simulink model "firstmodel"  (R2025a)
settings: Solver=FixedStepAuto  StartTime=0.0  StopTime=1  FixedStep=0.001  RelTol=1e-3
undefined symbols (not defined in the file): DiscIntNeverNeededParam
settings Model: Creator=DELL  LastModifiedBy=DELL

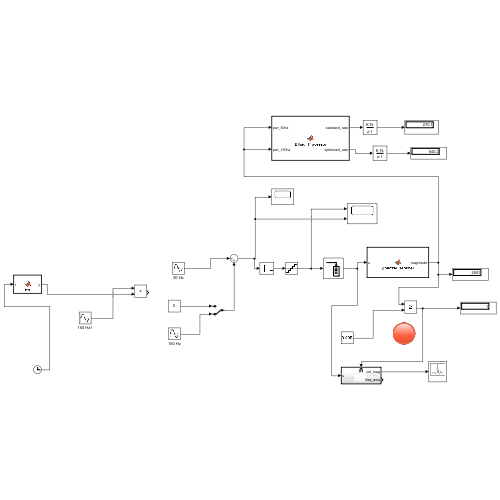
[thumbnail: Simulink's stored preview of the top-level diagram]
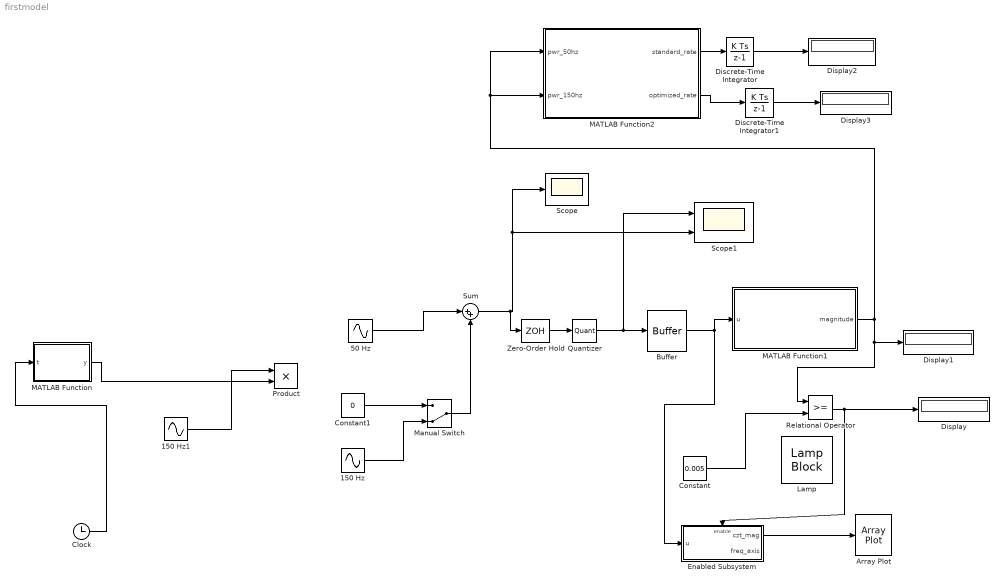
== system firstmodel ==
  150 Hz : Sin  Frequency=300*pi  SampleTime=0
  150 Hz1 : Sin  Frequency=300*pi  SampleTime=0
  50 Hz : Sin  Frequency=100*pi  SampleTime=0
  Array Plot : ArrayPlot  WindowPosition=[134.000000,171.000000,800.000000,500.000000,]  ScopeFrameLocation=window  SampleIncrement=0.02  XOffset=140  YLimits=[3.4950518655331093 6.194518570220462]
      settings: OpenAtSimulationStart=off
  Buffer : Buffer  N=100  OutputFrames=off
  Clock : Clock
  Constant : Constant  Value=0.005
  Constant1 : Constant  Value=0
  Discrete-Time Integrator : DiscreteIntegrator  SampleTime=-1  ICPrevOutput=DiscIntNeverNeededParam  ICPrevScaledInput=DiscIntNeverNeededParam
  Discrete-Time Integrator1 : DiscreteIntegrator  SampleTime=-1  ICPrevOutput=DiscIntNeverNeededParam  ICPrevScaledInput=DiscIntNeverNeededParam
  Display{,1..3} (4 alike) : Display
  Enabled Subsystem : Subsystem  TreatAsAtomicUnit=on
  Lamp : LampBlock  LabelPosition=Hide  DefaultColor=[192.0, 192.0, 192.0]
  MATLAB Function : MATLAB Function  TreatAsAtomicUnit=on
  MATLAB Function1 : MATLAB Function  TreatAsAtomicUnit=on
  MATLAB Function2 : MATLAB Function  TreatAsAtomicUnit=on
  Manual Switch : ManualSwitch  CurrentSetting=0
  Product : Product
  Quantizer : Quantizer  QuantizationInterval=2/4096
  Relational Operator : RelationalOperator  OutDataTypeStr=boolean  RndMeth=Simplest  InputSameDT=off
  Scope : Scope
      settings: ActiveDisplayYMinimum=-1.6931778606615959  ActiveDisplayYMaximum=1.933966715724176
  Scope1 : Scope  NumInputPorts=2
      settings: ActiveDisplayYMinimum=-1.923828125  ActiveDisplayYMaximum=1.923828125
  Sum : Sum  Inputs=|++
  Zero-Order Hold : ZeroOrderHold  SampleTime=1/1000
  wires:
  50 Hz/1 -> Sum/1
  Sum/1 -> Scope/1, Scope1/2, Zero-Order Hold/1
  Clock/1 -> MATLAB Function/1(t)
  MATLAB Function/1(y) -> Product/2
  Zero-Order Hold/1 -> Quantizer/1
  Quantizer/1 -> Buffer/1, Scope1/1
  Buffer/1 -> Enabled Subsystem/1(u), MATLAB Function1/1(u)
  MATLAB Function1/1(magnitude) -> MATLAB Function2/2(pwr_150hz), MATLAB Function2/1(pwr_50hz), Display1/1, Relational Operator/1
  Constant/1 -> Relational Operator/2
  Relational Operator/1 -> Display/1, Enabled Subsystem/Enable
  Constant1/1 -> Manual Switch/1
  150 Hz/1 -> Manual Switch/2
  Enabled Subsystem/1(czt_mag) -> Array Plot/1
  150 Hz1/1 -> Product/1
  MATLAB Function2/1(standard_rate) -> Discrete-Time Integrator/1
  Manual Switch/1 -> Sum/2
  MATLAB Function2/2(optimized_rate) -> Discrete-Time Integrator1/1
  Discrete-Time Integrator/1 -> Display2/1
  Discrete-Time Integrator1/1 -> Display3/1

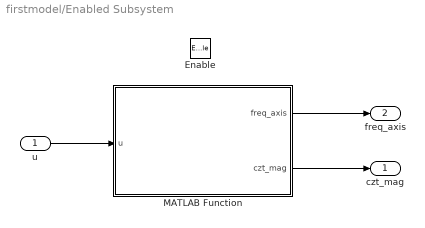
== system firstmodel/Enabled Subsystem ==
  u : Inport
  Enable : EnablePort
  MATLAB Function : MATLAB Function  TreatAsAtomicUnit=on
  czt_mag : Outport
  freq_axis : Outport  Port=2
  wires:
  u/1 -> MATLAB Function/1(u)
  MATLAB Function/1(freq_axis) -> freq_axis/1
  MATLAB Function/2(czt_mag) -> czt_mag/1

== matlab function firstmodel/MATLAB Function1 ==
  data: u input; magnitude output
function magnitude = goertzel_sentinel(u)
    % Parameters
    fs = 1000;          % Sampling frequency (1 kHz)
    f_target = 150;     % We are looking for the 3rd harmonic
    N = 100;            % Block size (number of samples to analyze)
    
    % Pre-calculate constants
    k = (N * f_target) / fs;
    w = (2 * pi / N) * k;
    coeff = 2 * cos(w);
    
    % Initialize states (these persist across samples if using global, 
    % but here we process a buffer for simplicity)
    s_prev1 = 0;
    s_prev2 = 0;
    
    % Recursive Goertzel Formula (from your PDF)
    for i = 1:length(u)
        s = u(i) + coeff * s_prev1 - s_prev2;
        s_prev2 = s_prev1;
        s_prev1 = s;
    end
    
    % Calculate Final Magnitude Power
    magnitude = s_prev2^2 + s_prev1^2 - coeff * s_prev1 * s_prev2;
end

== matlab function firstmodel/MATLAB Function ==
  data: t input; y output
function y = fcn(t)
% Tampering occurs between 20-40 seconds
if t >= 0.1 && t < 0.3
    y = 1;  % Attack ON
else
    y = 0;  % Attack OFF
end

== matlab function firstmodel/Enabled Subsystem/MATLAB Function ==
  data: u input; freq_axis output; czt_mag output
function [freq_axis, czt_mag] = czt_microscope(u)
    % Parameters from project specs
    fs = 1000;          % Sampling frequency
    f1 = 140;           % Start of zoom band 
    f2 = 160;           % End of zoom band 
    m = 1000;           % Resolution (1000 bins) 
    
    % Define the spiral contour parameters for CZT [cite: 72]
    w = exp(-1j * 2 * pi * (f2 - f1) / (m * fs));
    a = exp(1j * 2 * pi * f1 / fs);
    
    % Execute Chirp-Z Transform
    czt_output = czt(u, m, w, a);
    
    % Output data for visualization
    czt_mag = abs(czt_output);
    freq_axis = linspace(f1, f2, m);
end

== matlab function firstmodel/MATLAB Function2 ==
  data: pwr_50hz input; standard_rate output; pwr_150hz input; optimized_rate output
function [standard_rate, optimized_rate] = Billing_Processor(pwr_50hz, pwr_150hz)
    % Define your Unit Price here
    unit_price = 0.12; % Example: $0.12 per unit
    
    % 1. Clean up noise
    if pwr_150hz < 0.001 
        pwr_150hz = 0; 
    end
    
    % 2. Calculate Power Rates multiplied by Price
    % Note: These are still "Rates". They must be integrated in Simulink 
    % to become a "Bill" that grows over time.
    standard_rate = pwr_50hz * unit_price;
    optimized_rate = (pwr_50hz + pwr_150hz) * unit_price;
end
